simulink model "respuesta_seno"  (R2025a)
settings: Solver=VariableStepAuto  StartTime=0.0  StopTime=.2  RelTol=1e-3
values from neighbouring files (symbols this model uses):
  plant_c = ss([A+E*C],[B E],C,D)    [parametros_micro.m]
  Ts = 1e-5    (= 1e-05)    [der_delay_mpc.m]    (also in der_mpc.m; der_mpc_acoplado.m; parametros_micro.m = 5e-05; parametros_micro2.m = 5e-05)
settings Model: Creator=cmparedesv  LastModifiedBy=cmparedesv

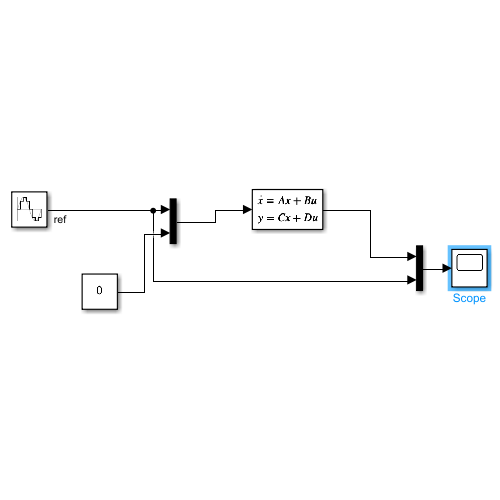
[thumbnail: Simulink's stored preview of the top-level diagram]
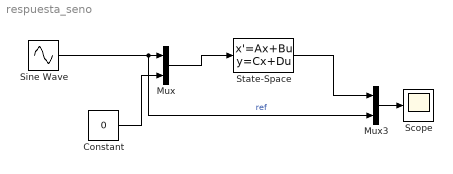
== system respuesta_seno ==
  Constant : Constant  Value=0
  Mux : Mux  Inputs=2
  Mux3 : Mux  Inputs=2
  Scope : Scope
      settings: ActiveDisplayYMinimum=-212.13203435608739  ActiveDisplayYMaximum=212.13203435601696
  Sine Wave : Sin  Amplitude=130*sqrt(2)  Frequency=2*pi*60  SampleTime=Ts
  State-Space : StateSpace  A=plant_c.A  B=plant_c.B  C=plant_c.C  D=plant_c.D  InitialCondition=0
  wires:
  Mux3/1 -> Scope/1
  State-Space/1 -> Mux3/1
  Mux/1 -> State-Space/1
  Sine Wave/1 -> Mux3/2, Mux/1  "ref"
  Constant/1 -> Mux/2
